simulink model "Vrabie"  (R2014b)
settings: Solver=ode45  StartTime=0.0  StopTime=5  FixedStep=0.0001  MaxStep=0.001  RelTol=1e-10  AbsTol=1e-10
InitFcn:
  | initializer
values from neighbouring files (symbols this model uses):
  A = [-.0665, 11.5, 0, 0 ... (first row only)    [initializer.m]
  B = [0; 0; 13.736; 0]    [initializer.m]
  C = eye(4)    [initializer.m]
  D = zeros(4,1)    [initializer.m]
  K_nom = R\B'*P_nom    [initializer.m]
  N = 20    [initializer.m]
  Q = eye(4)    [initializer.m]
  R = eye(1)    [initializer.m]
  start = floor((size(x_sim.Data, 1)-2)/N) * N + 1    [debug.m]    (also in initializer.m = 2)
  T = 0.05    [initializer.m]
  x0 = [0; 1e-1; 0; 0]    [initializer.m]
libraries: simulink x1
settings Model: Creator=Joseph  LastModifiedBy=Joseph

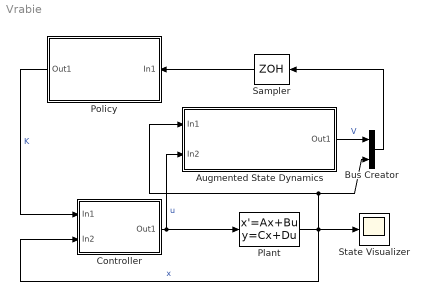
== system Vrabie ==
  Augmented State Dynamics : Subsystem
      mask Display:
      | port_label('input',1,'x','texmode','on');
      | port_label('input',2,'u','texmode','on');
      | port_label('output',1,'V','texmode','on');
      | disp('dV/dt = x^TQx + u^TRu','texmode','on');
  Bus Creator : BusCreator  Inputs=2
  Controller : Subsystem
      mask Display:
      | port_label('input',1,'K','texmode','on');
      | port_label('input',2,'x','texmode','on');
      | port_label('output',1,'u','texmode','on');
      | disp('u = -Kx','texmode','on');
  Plant : StateSpace  A=A  B=B  C=C  D=D  X0=x0
  Policy : Subsystem  mask{N=N, start=start, R=R, B=B}
      mask prompts: N "Number of measurements"; start "Measurement start"
      mask Display:
      | port_label('input',1,'[x; V]','texmode','on');
      | port_label('output',1,'K','texmode','on');
      | disp('Critic','texmode','on');
  Sampler : ZeroOrderHold  SampleTime=T
  State Visualizer : Scope
      settings: TimeRange=1  YMin=-0.15  YMax=0.15  SaveName=xData  MaxDataPoints=50000
  wires:
  Plant/1 -> State Visualizer/1, Bus Creator/2, Augmented State Dynamics/1(In1), Controller/2(In2)  "x"
  Augmented State Dynamics/1(Out1) -> Bus Creator/1  "V"
  Bus Creator/1 -> Sampler/1
  Sampler/1 -> Policy/1(In1)
  Controller/1(Out1) -> Plant/1, Augmented State Dynamics/2(In2)  "u"
  Policy/1(Out1) -> Controller/1(In1)  "K"

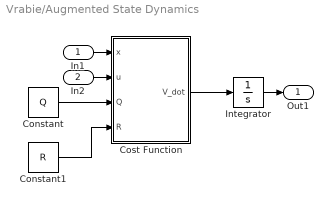
== system Vrabie/Augmented State Dynamics ==
  In1 : Inport
  In2 : Inport  Port=2
  Constant : Constant  Value=Q
  Constant1 : Constant  Value=R
  Cost Function : MATLAB Function  TreatAsAtomicUnit=on
  Integrator : Integrator
  Out1 : Outport
  wires:
  In1/1 -> Cost Function/1(x)
  Integrator/1 -> Out1/1
  Cost Function/1(V_dot) -> Integrator/1
  In2/1 -> Cost Function/2(u)
  Constant/1 -> Cost Function/3(Q)
  Constant1/1 -> Cost Function/4(R)

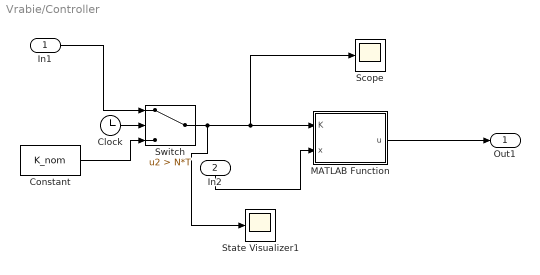
== system Vrabie/Controller ==
  In1 : Inport
  In2 : Inport  Port=2
  Clock : Clock
  Constant : Constant  Value=K_nom
  MATLAB Function : MATLAB Function  TreatAsAtomicUnit=on
  Scope : Scope
      settings: SaveName=ScopeData8
  State Visualizer1 : Scope
      settings: TimeRange=1  YMin=-0.15  YMax=0.15  SaveName=xData2  MaxDataPoints=50000
  Switch : Switch  Criteria=u2 > Threshold  Threshold=N*T
  Out1 : Outport
  wires:
  Clock/1 -> Switch/2
  Constant/1 -> Switch/3
  MATLAB Function/1(u) -> Out1/1
  In1/1 -> Switch/1
  In2/1 -> MATLAB Function/2(x)
  Switch/1 -> State Visualizer1/1, Scope/1, MATLAB Function/1(K)

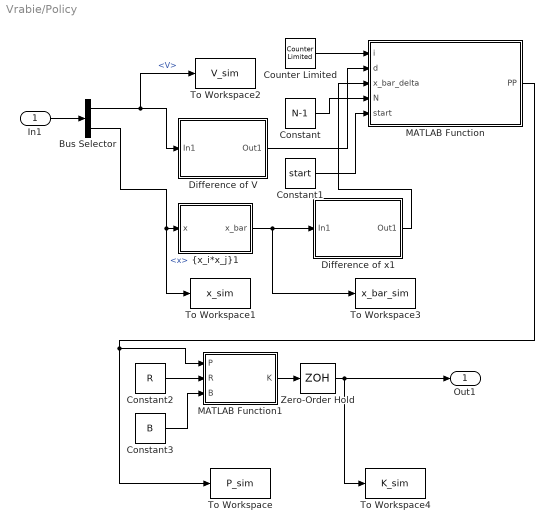
== system Vrabie/Policy ==
  In1 : Inport
  Bus Selector : BusSelector  OutputSignals=V,x
  Constant : Constant  Value=N-1
  Constant1 : Constant  Value=start
  Constant2 : Constant  Value=R
  Constant3 : Constant  Value=B
  Counter Limited : simulink/Sources/Counter Limited  uplimit=N-1  tsamp=-1
  Difference of V : Subsystem
      mask Display:
      | port_label('input',1,'V','texmode','on');
      | port_label('output',1,'d(x^i, K_i)','texmode','on');
  Difference of x1 : Subsystem
      mask Display:
      | port_label('input',1,'x','texmode','on');
      | port_label('output',1,'x_{\Delta}^i','texmode','on');
  MATLAB Function : MATLAB Function  TreatAsAtomicUnit=on  VariantControl=Variant1
  MATLAB Function1 : MATLAB Function  TreatAsAtomicUnit=on
  To Workspace : ToWorkspace  VariableName=P_sim  SaveFormat=Timeseries  SampleTime=-1
  To Workspace1 : ToWorkspace  VariableName=x_sim  SaveFormat=Timeseries  SampleTime=-1
  To Workspace2 : ToWorkspace  VariableName=V_sim  SaveFormat=Timeseries  SampleTime=-1
  To Workspace3 : ToWorkspace  VariableName=x_bar_sim  SaveFormat=Timeseries  SampleTime=-1
  To Workspace4 : ToWorkspace  VariableName=K_sim  SaveFormat=Timeseries  SampleTime=-1
  Zero-Order Hold : ZeroOrderHold  SampleTime=N*T
  "{x_i*x_j}1" : MATLAB Function  TreatAsAtomicUnit=on
  Out1 : Outport
  wires:
  Difference of x1/1(Out1) -> MATLAB Function/3(x_bar_delta)
  Difference of V/1(Out1) -> MATLAB Function/2(d)
  In1/1 -> Bus Selector/1
  Counter Limited/1 -> MATLAB Function/1(i)
  "{x_i*x_j}1"/1(x_bar) -> Difference of x1/1(In1), To Workspace3/1
  MATLAB Function/1(PP) -> MATLAB Function1/1(P), To Workspace/1
  Bus Selector/2 -> To Workspace1/1, "{x_i*x_j}1"/1(x)  "<x>"
  Bus Selector/1 -> To Workspace2/1, Difference of V/1(In1)  "<V>"
  Constant/1 -> MATLAB Function/4(N)
  Constant1/1 -> MATLAB Function/5(start)
  MATLAB Function1/1(K) -> Zero-Order Hold/1
  Constant2/1 -> MATLAB Function1/2(R)
  Constant3/1 -> MATLAB Function1/3(B)
  Zero-Order Hold/1 -> Out1/1, To Workspace4/1

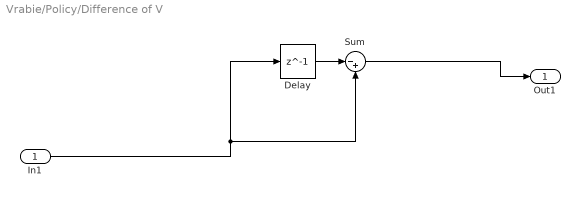
== system Vrabie/Policy/Difference of V ==
  In1 : Inport
  Delay : Delay  DelayLength=1  InitialCondition=0
  Sum : Sum  Inputs=|-+
  Out1 : Outport
  wires:
  Delay/1 -> Sum/1
  Sum/1 -> Out1/1
  In1/1 -> Sum/2, Delay/1

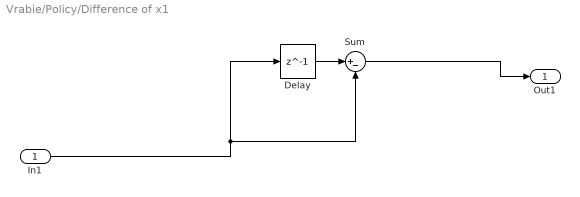
== system Vrabie/Policy/Difference of x1 ==
  In1 : Inport
  Delay : Delay  DelayLength=1  InitialCondition=0
  Sum : Sum  Inputs=|+-
  Out1 : Outport
  wires:
  In1/1 -> Delay/1, Sum/2
  Sum/1 -> Out1/1
  Delay/1 -> Sum/1

== matlab function Vrabie/Augmented State Dynamics/Cost Function ==
  data: x input; u input; V_dot output; Q input; R input
function V_dot = fcn(x, u, Q, R)
%#codegen

V_dot = x'*Q*x + u'*R*u;

== matlab function Vrabie/Policy/MATLAB Function1 ==
  data: P input; K output; R input; B input
function K = fcn(P, R, B)
K = R\B'*P;

== matlab function Vrabie/Policy/{x_i*x_j}1 ==
  data: x input; x_bar output
function x_bar = fcn(x)

n = size(x,1);
x_bar = zeros(n*(n+1)/2, 1);

count = 1;
for i=1:n
    for j=i:n
        x_bar(count) = x(i)*x(j);
        count = count + 1;
    end
end

== matlab function Vrabie/Policy/MATLAB Function ==
  data: i input; d input; PP output; x_bar_delta input; N input; start input
function PP = fcn(i, d, x_bar_delta, N, start)
persistent X Y P p_1 has_converged
if N > 200
%     N = 200;
    error('N is too big');
end
if start < 1
    error('start cannot be less than 1');
end
if N-start <10
    error('(N - start) must be greater than or equal to 10');
end
if isempty(X)
    X = zeros(10, N-start); 
end
if isempty(Y)
    Y = zeros(1, N-start);
end
if isempty(P)
    P = zeros(4,4);
end
if isempty(p_1)
    p_1 = zeros(10,1);
end
if isempty(has_converged)
    has_converged = false;
end

if i == 0
    X = zeros(10, N-start);
    Y = zeros(1, N-start);
elseif i >= start && i <= N-1
    X(:, i+1-start) = x_bar_delta;
    Y(:, i+1-start) = d;
end

if i == N-1 && has_converged == false
    p = (X*X')\X*Y';
    diff =  norm(p - p_1)/norm(p);
    if diff < 0.1
        has_converged = true;
    end
    p_1 = p;
    
    P = zeros(4,4);
    P(1:4,1) = p(1:4);
    P(2:4,2) = p(5:7);
    P(3:4,3) = p(8:9);
    P(4,4) = p(10);
    P = (P + P') / 2;
end

PP = P;

== matlab function Vrabie/Controller/MATLAB Function ==
  data: u output; K input; x input
function u = fcn(K, x)

u = -K'*x;
